simulink model "PositionPlantTest"  (R2020a)
settings: Solver=VariableStepAuto  StartTime=0.0  StopTime=10.0  RelTol=1e-3
settings Model: Creator=scott  LastModifiedBy=scott

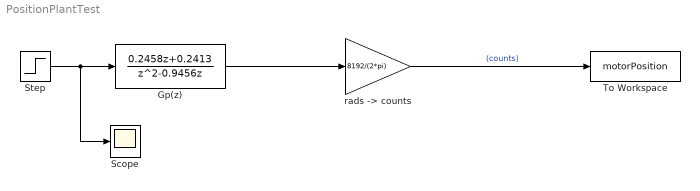
== system PositionPlantTest ==
  Gp(z) : DiscreteTransferFcn  Numerator=[0.2458 0.2413]  Denominator=[1 -0.9456 0]  SampleTime=0.008
  Scope : Scope
  Step : Step  Time=0  SampleTime=0
  To Workspace : ToWorkspace  VariableName=motorPosition  SaveFormat=Timeseries  SampleTime=-1
  "rads -> counts" : Gain  Gain=8192/(2*pi)
  wires:
  Gp(z)/1 -> "rads -> counts"/1
  "rads -> counts"/1 -> To Workspace/1  "(counts)"
  Step/1 -> Scope/1, Gp(z)/1
